simulink model "Motor_Pos_cl"  (Simulink 7.5)
settings: Solver=ode15s  StartTime=0.0  StopTime=0.08  RelTol=1e-3
undefined symbols (not defined in the file): b, J, K, L, R
settings Model: Creator=maen  LastModifiedBy=Rick
settings DebuggingCC: SolverPrmCheckMsg=none

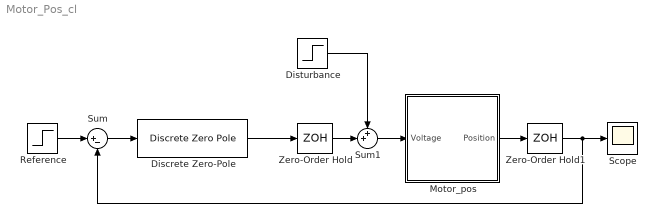
== system Motor_Pos_cl ==
  Discrete Zero-Pole : DiscreteZeroPole  Zeros=[0.95 0.80 0.80]  Poles=[-0.98 0.6 1]  Gain=800  SampleTime=0.001
  Disturbance : Step  Time=0.03  SampleTime=0
  Motor_pos : Subsystem
  Reference : Step  Time=0  SampleTime=0
  Scope : Scope
      settings: YMin=1.0025  YMax=1.04
  Sum : Sum  Inputs=|+-  OutDataType=fixdt(1, 16)  OutScaling=2^0
  Sum1 : Sum  Inputs=++|  OutDataType=fixdt(1, 16)  OutScaling=2^0
  Zero-Order Hold : ZeroOrderHold  SampleTime=0.001
  Zero-Order Hold1 : ZeroOrderHold  SampleTime=0.001
  wires:
  Zero-Order Hold1/1 -> Scope/1, Sum/2
  Sum/1 -> Discrete Zero-Pole/1
  Motor_pos/1(Position) -> Zero-Order Hold1/1
  Reference/1 -> Sum/1
  Discrete Zero-Pole/1 -> Zero-Order Hold/1
  Zero-Order Hold/1 -> Sum1/2
  Sum1/1 -> Motor_pos/1(Voltage)
  Disturbance/1 -> Sum1/1

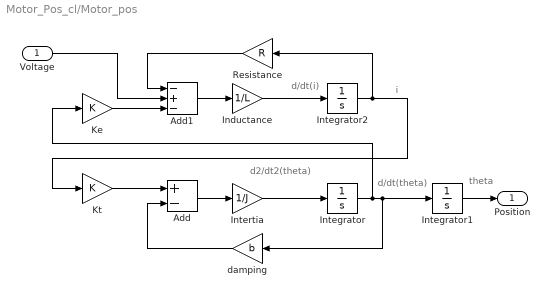
== system Motor_Pos_cl/Motor_pos ==
  note: i
  note: d/dt(theta)
  note: d2/dt2(theta)
  note: d/dt(i)
  note: theta
  Voltage : Inport  OutDataType=fixdt(1, 16)  OutScaling=2^0
  Add : Sum  Inputs=+-  OutDataType=fixdt(1, 16)  OutScaling=2^-10
  Add1 : Sum  Inputs=-+-  OutDataType=fixdt(1, 16)  OutScaling=2^-10
  Inductance : Gain  Gain=1/L  ParameterDataType=fixdt(1, 16)  ParameterScaling=2^0  OutDataType=fixdt(1, 16)  OutScaling=2^0
  Integrator : Integrator
  Integrator1 : Integrator
  Integrator2 : Integrator
  Intertia : Gain  Gain=1/J  ParameterDataType=fixdt(1, 16)  ParameterScaling=2^0  OutDataType=fixdt(1, 16)  OutScaling=2^0
  Ke : Gain  Gain=K  ParameterDataType=fixdt(1, 16)  ParameterScaling=2^0  OutDataType=fixdt(1, 16)  OutScaling=2^0
  Kt : Gain  Gain=K  ParameterDataType=fixdt(1, 16)  ParameterScaling=2^0  OutDataType=fixdt(1, 16)  OutScaling=2^0
  Resistance : Gain  Gain=R  ParameterDataType=fixdt(1, 16)  ParameterScaling=2^0  OutDataType=fixdt(1, 16)  OutScaling=2^0
  damping : Gain  Gain=b  ParameterDataType=fixdt(1, 16)  ParameterScaling=2^0  OutDataType=fixdt(1, 16)  OutScaling=2^0
  Position : Outport  OutDataType=fixdt(1, 16)  OutScaling=2^0
  wires:
  Inductance/1 -> Integrator2/1
  Integrator/1 -> Integrator1/1, damping/1, Ke/1
  Integrator1/1 -> Position/1
  Intertia/1 -> Integrator/1
  Integrator2/1 -> Kt/1, Resistance/1
  Add/1 -> Intertia/1
  Add1/1 -> Inductance/1
  Kt/1 -> Add/1
  damping/1 -> Add/2
  Ke/1 -> Add1/3
  Resistance/1 -> Add1/1
  Voltage/1 -> Add1/2
